simulink model "Sim_Modell_RFJ"  (R2020b)
settings: Solver=VariableStepAuto  StartTime=0.0  StopTime=10.0  RelTol=1e-3
undefined symbols (not defined in the file or in its folder): ACD120_80_Rotor, ACD120_80_Stator, Ausleger, Auslegerplatte, DistanzhuelseGP, Federbolzen, Grundplatte, Heidenhain_ERN_1080, Lagerdeckel_oben, Lagerdeckel_unten, par_imp, parSys, Seitenplatte, Visualisierung, Welle, X, Y, Z
libraries: sm_lib x37, fl_lib x7, nesl_utility x7, cstblocks x2, simulink x1
(part 3 of 3)

== matlab function Sim_Modell_RFJ/system (nonlinear)/MATLAB Function1 ==
  data: x input; y output; parSys parameter
function y = fcn(x, parSys)

y = zeros(3,1); % necesary for home

% map the states
phit=x(1);
phia=x(2);
omega=x(3);

% create the output
y(1) = phia;
y(2) = omega;
y(3) = phit;
